simulink model "ram_test"  (R2015a)
settings: Solver=FixedStepDiscrete  SolverMode=SingleTasking  StartTime=0.0  StopTime=10.0  FixedStep=1e-3  RelTol=1e-3
values from neighbouring files (symbols this model uses):
  Param1 = 1.0    [mbed_flash_constants.sldd]
undefined symbols (not defined in the file or in its folder): Param
libraries: mbed_targets_stm_disco_f407 x1
settings Model: DataDictionary=ram_test.sldd  Creator=Sandra  LastModifiedBy=oh
settings OptimizationCC: BlockReduction=off  InlineParams=on  OptimizeModelRefInitCode=on  LifeSpan=1
settings HardwareCC: ProdLargestAtomicInteger=Long  ProdLargestAtomicFloat=Double  ProdEndianess=LittleEndian  ProdHWDeviceType=ARM Compatible->ARM Cortex
settings RTWCC: SystemTargetFile=mbed.tlc  TemplateMakefile=mbed.tmf  Description=Mbed Target (Embedded Target)  GenerateReport=on  IncludeHyperlinkInReport=on  LaunchReport=on  TargetLang=C++  GenerateTraceInfo=on  GenerateTraceReport=on  GenerateTraceReportSl=on  GenerateTraceReportSf=on  GenerateTraceReportEml=on
settings CodeAppCC: IgnoreCustomStorageClasses=off
settings STFCustomTargetCC: CombineOutputUpdateFcns=on  SupportContinuousTime=off  SupportVariableSizeSignals=off  SystemTargetFile=mbed.tlc
settings ERTTargetCC: SupportContinuousTime=off  SupportVariableSizeSignals=off  ERTCustomFileTemplate=mbed_file_process.tlc  MemSecPackage=mbed_csc

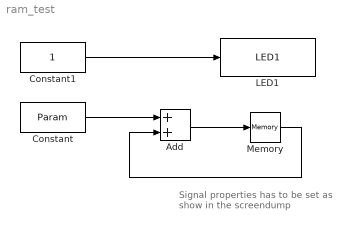
== system ram_test ==
  note: Signal properties has to be
      | set as show in the screendump
  Add : Sum
  Constant : Constant  Value=Param
  Constant1 : Constant  OutDataTypeStr=uint8
  LED1 : mbed_targets_stm_disco_f407/LED1  Parameter1=0
  Memory : Memory  X0=Param1  StateIdentifier=Sig
      settings: AttributesFormatString=%<X0>
  wires:
  Add/1 -> Memory/1
  Memory/1 -> Add/2
  Constant1/1 -> LED1/1
  Constant/1 -> Add/1
